simulink model "chap8_3sim"  (Simulink 8.1)
settings: Solver=ode45  StartTime=0.0  StopTime=30  RelTol=1e-3
settings Model: Creator=Administrator  LastModifiedBy=liujk
settings DataIOCC: SignalLoggingName=sigsOut
settings OptimizationCC: InitFltsAndDblsToZero=on
settings DebuggingCC: SaveWithParameterizedLinksMsg=none  SignalResolutionControl=TryResolveAllWithWarning  SolverPrmCheckMsg=none  MultiTaskDSMMsg=warning  MultiTaskCondExecSysMsg=none  StrictBusMsg=None
settings HardwareCC: TargetUnknown=on
settings RTWCC: IncludeERTFirstTime=on
settings GRTTargetCC: TargetFcnLib=ansi_tfl_tmw.mat

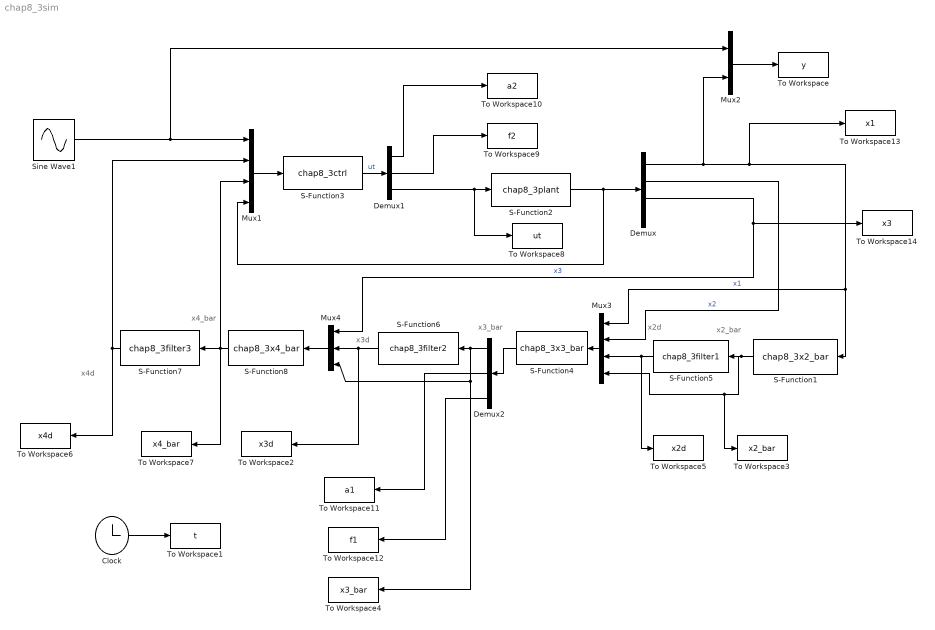
== system chap8_3sim ==
  note: x2d
  note: x2_bar
  note: x3_bar
  note: x3d
  note: x4_bar
  note: x4d
  Clock : Clock
  Demux : Demux
  Demux1 : Demux  Outputs=3
  Demux2 : Demux  Outputs=3
  Mux1 : Mux
  Mux2 : Mux  Inputs=2
  Mux3 : Mux
  Mux4 : Mux  Inputs=3
  S-Function1 : S-Function  FunctionName=chap8_3x2_bar  EnableBusSupport=off
  S-Function2 : S-Function  FunctionName=chap8_3plant  EnableBusSupport=off
  S-Function3 : S-Function  FunctionName=chap8_3ctrl  EnableBusSupport=off
  S-Function4 : S-Function  FunctionName=chap8_3x3_bar  EnableBusSupport=off
  S-Function5 : S-Function  FunctionName=chap8_3filter1  EnableBusSupport=off
  S-Function6 : S-Function  FunctionName=chap8_3filter2  EnableBusSupport=off
  S-Function7 : S-Function  FunctionName=chap8_3filter3  EnableBusSupport=off
  S-Function8 : S-Function  FunctionName=chap8_3x4_bar  EnableBusSupport=off
  Sine Wave1 : Sin  SampleTime=0
  To Workspace : ToWorkspace  VariableName=y  SampleTime=-1
  To Workspace1 : ToWorkspace  VariableName=t  SampleTime=-1
  To Workspace10 : ToWorkspace  VariableName=a2  SampleTime=-1
  To Workspace11 : ToWorkspace  VariableName=a1  SampleTime=-1
  To Workspace12 : ToWorkspace  VariableName=f1  SampleTime=-1
  To Workspace13 : ToWorkspace  VariableName=x1  SampleTime=-1
  To Workspace14 : ToWorkspace  VariableName=x3  SampleTime=-1
  To Workspace2 : ToWorkspace  VariableName=x3d  SampleTime=-1
  To Workspace3 : ToWorkspace  VariableName=x2_bar  SampleTime=-1
  To Workspace4 : ToWorkspace  VariableName=x3_bar  SampleTime=-1
  To Workspace5 : ToWorkspace  VariableName=x2d  SampleTime=-1
  To Workspace6 : ToWorkspace  VariableName=x4d  SampleTime=-1
  To Workspace7 : ToWorkspace  VariableName=x4_bar  SampleTime=-1
  To Workspace8 : ToWorkspace  VariableName=ut  SampleTime=-1
  To Workspace9 : ToWorkspace  VariableName=f2  SampleTime=-1
  wires:
  Clock/1 -> To Workspace1/1
  Mux1/1 -> S-Function3/1
  Sine Wave1/1 -> Mux2/1, Mux1/1
  S-Function2/1 -> Demux/1, Mux1/4
  Demux/1 -> Mux2/2, Mux3/1, S-Function1/1, To Workspace13/1  "x1"
  Mux2/1 -> To Workspace/1
  Mux3/1 -> S-Function4/1
  Demux/3 -> Mux4/1, To Workspace14/1  "x3"
  S-Function1/1 -> To Workspace3/1, Mux3/4, S-Function5/1
  S-Function8/1 -> To Workspace7/1, S-Function7/1, Mux1/3
  Mux4/1 -> S-Function8/1
  S-Function6/1 -> Mux4/2, To Workspace2/1
  S-Function7/1 -> To Workspace6/1, Mux1/2
  S-Function5/1 -> Mux3/3, To Workspace5/1
  Demux/2 -> Mux3/2  "x2"
  S-Function3/1 -> Demux1/1  "ut"
  Demux1/3 -> S-Function2/1, To Workspace8/1
  Demux1/1 -> To Workspace10/1
  Demux1/2 -> To Workspace9/1
  S-Function4/1 -> Demux2/1
  Demux2/1 -> S-Function6/1, Mux4/3, To Workspace4/1
  Demux2/2 -> To Workspace11/1
  Demux2/3 -> To Workspace12/1
